simulink model "LaoWang_chap10_calibration"  (R2022a)
settings: Solver=VariableStepAuto  StartTime=0.0  StopTime=50  RelTol=1e-3
undefined symbols (not defined in the file or in its folder): au, table, thr, vu
libraries: Solver_SF x1
settings Model: Creator=wwcong  LastModifiedBy=HaiChen
settings SolverCC: AlgebraicLoopSolver=TrustRegion
settings DataIOCC: ReturnWorkspaceOutputs=off
settings DebuggingCC: UnconnectedInputMsg=warning  UnconnectedOutputMsg=warning  UnconnectedLineMsg=warning  SFMachineParentedDataDiag=warning  ArithmeticOperatorsInVariantConditions=warning
settings SFSimCC: SimUseLocalCustomCode=off  CustomCodeUndefinedFunction=UseInterfaceOnly
settings RTWCC: RTWUseLocalCustomCode=off

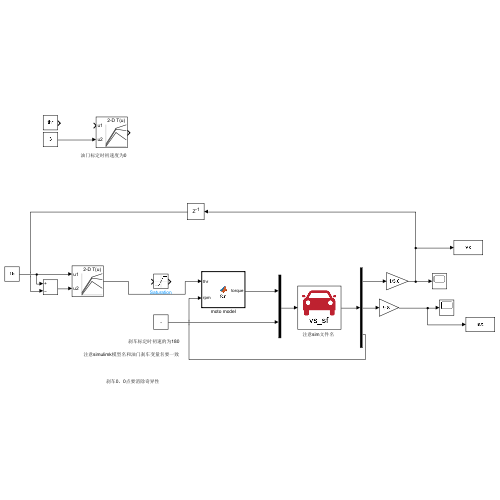
[thumbnail: Simulink's stored preview of the top-level diagram]
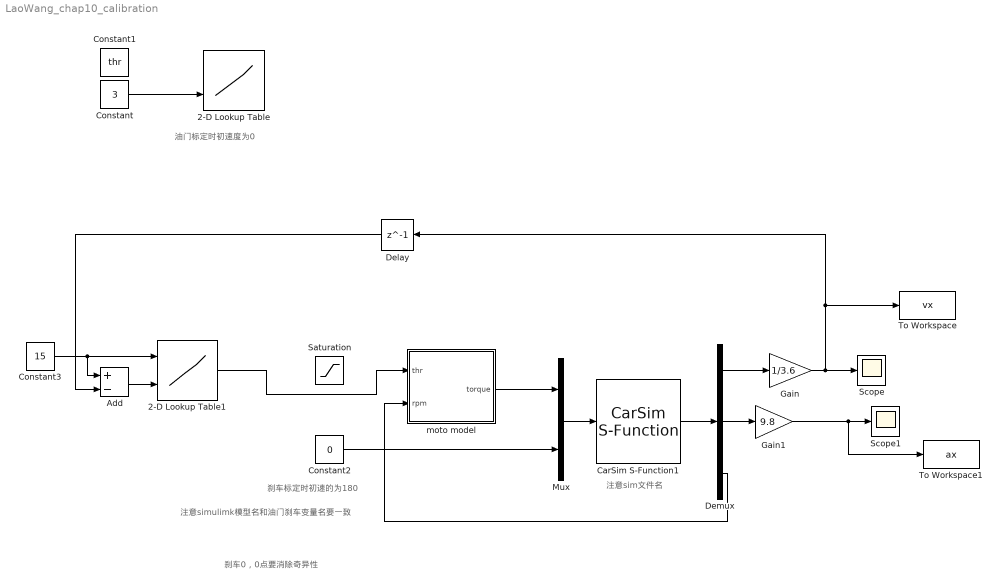
== system LaoWang_chap10_calibration ==
  note: 刹车0，0点要消除奇异性
  note: 注意simulimk模型名和油门刹车变量名要一致
  note: 刹车标定时初速的为180
  note: 油门标定时初速度为0
  note: 注意sim文件名
  2-D Lookup Table : Lookup_n-D  BreakpointsForDimension1=vu  BreakpointsForDimension2=au  Table=table  InternalRulePriority=Speed  RndMeth=Simplest
      settings: InputPortMap=u0,u1
  2-D Lookup Table1 : Lookup_n-D  BreakpointsForDimension1=vu  BreakpointsForDimension2=au  Table=table  InternalRulePriority=Speed  RndMeth=Simplest
      settings: InputPortMap=u0,u1
  Add : Sum  Inputs=+-
  CarSim S-Function1 : Solver_SF/CarSim S-Function  Priority=1  SIMFILE=LaoWang_chap10_calibration.sim
  Constant : Constant  Value=3
  Constant1 : Constant  Value=thr
  Constant2 : Constant  Value=0
  Constant3 : Constant  Value=15
  Delay : Delay  DelayLength=1
  Demux : Demux  Outputs=3
  Gain : Gain  Gain=1/3.6
  Gain1 : Gain  Gain=9.8
  Mux : Mux  Inputs=2
  Saturation : Saturate  UpperLimit=1
  Scope : Scope
  Scope1 : Scope
  To Workspace : ToWorkspace  VariableName=vx  SaveFormat=Timeseries  SampleTime=0.1
  To Workspace1 : ToWorkspace  VariableName=ax  SaveFormat=Timeseries  SampleTime=0.1
  moto model : MATLAB Function  TreatAsAtomicUnit=on
  wires:
  Mux/1 -> CarSim S-Function1/1
  CarSim S-Function1/1 -> Demux/1
  Demux/1 -> Gain/1
  Demux/2 -> Gain1/1
  Gain1/1 -> Scope1/1, To Workspace1/1
  Gain/1 -> To Workspace/1, Delay/1, Scope/1
  Demux/3 -> moto model/2(rpm)
  moto model/1(torque) -> Mux/1
  Constant2/1 -> Mux/2
  Constant/1 -> 2-D Lookup Table/2
  Constant3/1 -> Add/1, 2-D Lookup Table1/1
  Add/1 -> 2-D Lookup Table1/2
  Delay/1 -> Add/2
  2-D Lookup Table1/1 -> moto model/1(thr)

== matlab function LaoWang_chap10_calibration/moto model ==
  data: thr input; torque output; rpm input
function torque = fcn(thr,rpm)
Tmax=380*thr;
    if (rpm<=4523)
        torque=Tmax;
    else
        torque=Tmax*4523/rpm;
    end
end
